simulink model "RadarSimulink"  (R2024b)
settings: Solver=VariableStepAuto  StartTime=0.0  StopTime=20  RelTol=1e-3
values from neighbouring files (symbols this model uses):
  R = mn^2    (= 2500)    [RadarTracker.m]
undefined symbols (not defined in the file or in its folder): Discrete, Time
libraries: ctrlSharedLib x1
settings Model: Creator=John Schatzel  LastModifiedBy=John Schatzel

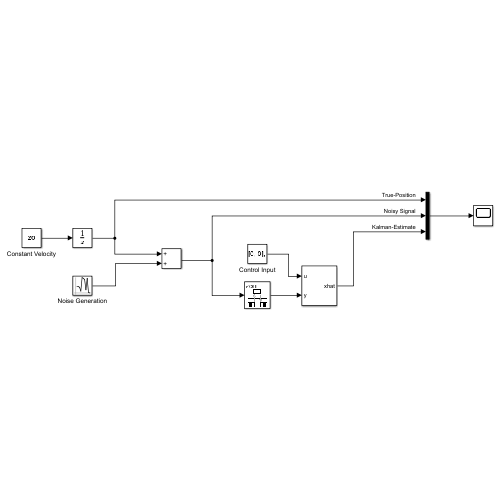
[thumbnail: Simulink's stored preview of the top-level diagram]
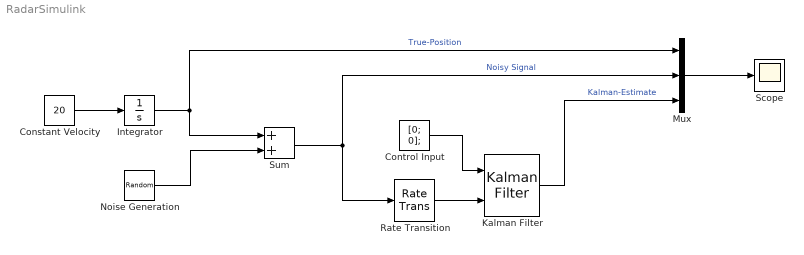
== system RadarSimulink ==
  Constant Velocity : Constant  Value=20
  Control Input : Constant  Value=[0; 0];
  Integrator : Integrator
  Kalman Filter : ctrlSharedLib/Kalman Filter  TimeDomain=Discrete-Time  UseCurrentEstimator=on  ModelSource=LTI State-Space Variable  ModelSourceVariable=sys  A=0.95  B=1  C=1  D=0  NumberOfStates=1  NumberOfInputs=1  NumberOfOutputs=1  InitialEstimateSource=Dialog  X0=[0; 0]  P0=10  UseK=off  UseGH=off  NumberOfProcessNoiseInputs=1  G=1  TimeInvariantG=on  H=0  TimeInvariantH=on  Q=Q  TimeInvariantQ=on  R=R  TimeInvariantR=on  N=0  TimeInvariantN=on  AddInputPort=on  AddEnablePort=off  OutputEstimatedY=off  OutputP=off  Ts=-1
  Mux : Mux  Inputs=3
  Noise Generation : RandomNumber  Variance=R  SampleTime=0.25  VectorParams1D=off
  Rate Transition : RateTransition  OutPortSampleTime=0.25
  Scope : Scope
  Sum : Sum
  wires:
  Constant Velocity/1 -> Integrator/1
  Integrator/1 -> Mux/1, Sum/1  "True-Position"
  Noise Generation/1 -> Sum/2
  Sum/1 -> Rate Transition/1, Mux/2  "Noisy Signal"
  Mux/1 -> Scope/1
  Control Input/1 -> Kalman Filter/1
  Rate Transition/1 -> Kalman Filter/2
  Kalman Filter/1 -> Mux/3  "Kalman-Estimate"
